simulink model "gm_Model"  (R2025a)
settings: Solver=FixedStepDiscrete  StartTime=0.0  StopTime=80000/fs_in  RelTol=1e-3
undefined symbols (not defined in the file or in its folder): a, b, b_fixp, beta_retanh, c, cos_omega, cos_omega_fixp, diag_count, exp_omega, exp_omega_fixp, fixp_chebacc_frac, fixp_chebacc_ws, fixp_dsp_ws, fixp_eig_frac, fixp_eig_ws, fs_in, group_size, hann_table_fixp, image_seed, image_seed_fixp, J_ROM, k, K_ROM, lap_diags, lap_main, lap_main_fi, lap_offsets, lap_offsets_fi, lap_rest, lap_rest_fi, laplacian_diags_main, laplacian_diags_offsets, laplacian_diags_rest, lut_norm_x, lut_norm_y, magnitude, n_ch, n_layer, n_px, n_px_fi, nf, norm_gain_floor, power_iters, power_norm_scaling_factor_fixp, tau, tau_fixp, theta, theta_fixp
libraries: simulink x59, hdlsllib x36, hdlstreaminglib x4, hdlmdlgenlib x1, matrix_library x1, dspvision x1
(part 3 of 8)

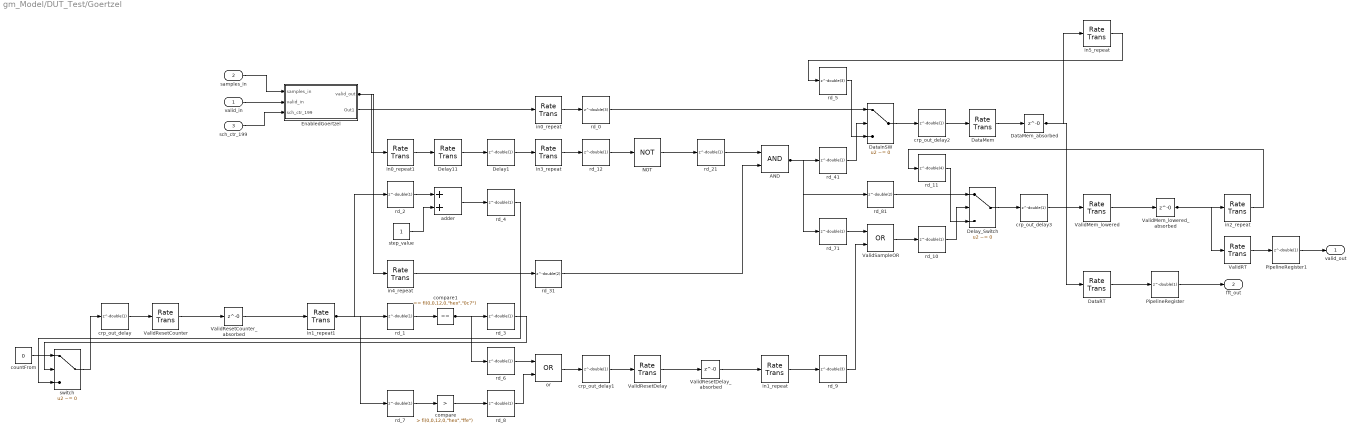
== system gm_Model/DUT_Test/Goertzel ==
  valid_in : Inport  OutDataTypeStr=boolean  PortDimensions=1  SampleTime=6.25e-05
  samples_in : Inport  Port=2  OutDataTypeStr=fixdt(1, 12, 11)  PortDimensions=[1 48]  SampleTime=6.25e-05
  sch_ctr_199 : Inport  Port=3  OutDataTypeStr=uint8  SampleTime=3.125e-07
  AND : Logic  AllPortsSameDT=off  OutDataTypeStr=boolean  SampleTime=3.125e-07
  DataInSW : Switch  Criteria=u2 ~= 0  Threshold="fi(0,0,1,0,\"hex\",\"0\")"  OutDataTypeStr=fixdt(1, 18, 13)  SampleTime=3.125e-07  SaturateOnIntegerOverflow=off  InputSameDT=off
  DataMem : RateTransition  InitialCondition=double(0)  OutPortSampleTimeOpt=Multiple of input port sample time  OutPortSampleTimeMultiple=200
  DataMem_absorbed : Delay  DelayLength=0
  DataRT : RateTransition  InitialCondition=double(0)  OutPortSampleTimeOpt=Multiple of input port sample time  OutPortSampleTimeMultiple=200
  Delay1 : Delay  DelayLength=double(1)  InitialCondition=0  SampleTime=6.25e-05
  Delay11 : RateTransition  InitialCondition=double(0)  OutPortSampleTimeOpt=Multiple of input port sample time  OutPortSampleTimeMultiple=200
  Delay_Switch : Switch  Criteria=u2 ~= 0  Threshold=double(0)  OutDataTypeStr=boolean  SampleTime=3.125e-07  SaturateOnIntegerOverflow=off  InputSameDT=off
  EnabledGoertzel : Subsystem
  NOT : Logic  Operator=NOT  Inputs=1  AllPortsSameDT=off  OutDataTypeStr=boolean  SampleTime=3.125e-07
  PipelineRegister : Delay  DelayLength=double(1)  InitialCondition=0  SampleTime=0.0125
  PipelineRegister1 : Delay  DelayLength=double(1)  InitialCondition=0  SampleTime=0.0125
  ValidMem_lowered : RateTransition  InitialCondition=double(0)  OutPortSampleTimeOpt=Multiple of input port sample time  OutPortSampleTimeMultiple=200
  ValidMem_lowered_absorbed : Delay  DelayLength=0
  ValidRT : RateTransition  InitialCondition=double(0)  OutPortSampleTimeOpt=Multiple of input port sample time  OutPortSampleTimeMultiple=200
  ValidResetCounter : RateTransition  InitialCondition=double(0)  OutPortSampleTimeOpt=Multiple of input port sample time  OutPortSampleTimeMultiple=200
  ValidResetCounter_absorbed : Delay  DelayLength=0
  ValidResetDelay : RateTransition  InitialCondition=double(0)  OutPortSampleTimeOpt=Multiple of input port sample time  OutPortSampleTimeMultiple=200
  ValidResetDelay_absorbed : Delay  DelayLength=0
  ValidSampleOR : Logic  Operator=OR  AllPortsSameDT=off  OutDataTypeStr=boolean  SampleTime=3.125e-07
  adder : Sum  OutDataTypeStr=fixdt(0, 12, 0)  AccumDataTypeStr=fixdt(0, 12, 0)  SampleTime=3.125e-07
  compare : simulink/Logic and Bit Operations/Compare To Constant  relop=>  const="fi(0,0,12,0,\"hex\",\"ffe\")"  OutDataTypeStr=boolean
  compare1 : simulink/Logic and Bit Operations/Compare To Constant  relop===  const="fi(0,0,12,0,\"hex\",\"0c7\")"  OutDataTypeStr=boolean
  countFrom : Constant  Value=0  VectorParams1D=off  OutDataTypeStr=fixdt(0, 12, 0)  SampleTime=3.125e-07
  crp_out_delay{,1..3} (4 alike) : Delay  DelayLength=double(1)  InitialCondition=0  SampleTime=3.125e-07
  in0_repeat : RateTransition  Integrity=off  Deterministic=off  OutPortSampleTimeOpt=Multiple of input port sample time  OutPortSampleTimeMultiple=1/200
  in0_repeat1 : RateTransition  Integrity=off  Deterministic=off  OutPortSampleTimeOpt=Multiple of input port sample time  OutPortSampleTimeMultiple=1/200
  in1_repeat : RateTransition  Integrity=off  Deterministic=off  OutPortSampleTimeOpt=Multiple of input port sample time  OutPortSampleTimeMultiple=1/200
  in1_repeat1 : RateTransition  Integrity=off  Deterministic=off  OutPortSampleTimeOpt=Multiple of input port sample time  OutPortSampleTimeMultiple=1/200
  in2_repeat : RateTransition  Integrity=off  Deterministic=off  OutPortSampleTimeOpt=Multiple of input port sample time  OutPortSampleTimeMultiple=1/200
  in3_repeat : RateTransition  Integrity=off  Deterministic=off  OutPortSampleTimeOpt=Multiple of input port sample time  OutPortSampleTimeMultiple=1/200
  in4_repeat : RateTransition  Integrity=off  Deterministic=off  OutPortSampleTimeOpt=Multiple of input port sample time  OutPortSampleTimeMultiple=1/200
  in5_repeat : RateTransition  Integrity=off  Deterministic=off  OutPortSampleTimeOpt=Multiple of input port sample time  OutPortSampleTimeMultiple=1/200
  or : Logic  Operator=OR  AllPortsSameDT=off  OutDataTypeStr=boolean  SampleTime=3.125e-07
  rd_0 : Delay  DelayLength=double(3)  InitialCondition=0  SampleTime=3.125e-07
  rd_{1..4,6..8,10,12,21,41,71} (12 alike) : Delay  DelayLength=double(1)  InitialCondition=0  SampleTime=3.125e-07
  rd_11 : Delay  DelayLength=double(4)  InitialCondition=0  SampleTime=3.125e-07
  rd_31 : Delay  DelayLength=double(2)  InitialCondition=0  SampleTime=3.125e-07
  rd_5 : Delay  DelayLength=double(3)  InitialCondition=0  SampleTime=3.125e-07
  rd_81 : Delay  DelayLength=double(2)  InitialCondition=0  SampleTime=3.125e-07
  rd_9 : Delay  DelayLength=double(3)  InitialCondition=0  SampleTime=3.125e-07
  step_value : Constant  VectorParams1D=off  OutDataTypeStr=fixdt(0, 12, 0)  SampleTime=3.125e-07
  switch : Switch  Criteria=u2 ~= 0  Threshold="fi(0,0,1,0,\"hex\",\"0\")"  OutDataTypeStr=fixdt(0, 12, 0)  SampleTime=3.125e-07  SaturateOnIntegerOverflow=off  InputSameDT=off
  valid_out : Outport  SampleTime=0.0125
  fft_out : Outport  Port=2  SampleTime=0.0125
  wires:
  valid_in/1 -> EnabledGoertzel/2(valid_in)
  countFrom/1 -> switch/1
  ValidResetDelay_absorbed/1 -> in1_repeat/1
  adder/1 -> rd_4/1
  switch/1 -> crp_out_delay/1
  in5_repeat/1 -> rd_5/1
  in1_repeat1/1 -> rd_2/1, rd_1/1, rd_7/1
  crp_out_delay/1 -> ValidResetCounter/1
  DataMem/1 -> DataMem_absorbed/1
  ValidResetCounter_absorbed/1 -> in1_repeat1/1
  DataMem_absorbed/1 -> DataRT/1, in5_repeat/1
  ValidResetCounter/1 -> ValidResetCounter_absorbed/1
  rd_0/1 -> DataInSW/1
  samples_in/1 -> EnabledGoertzel/1(samples_in)
  sch_ctr_199/1 -> EnabledGoertzel/3(sch_ctr_199)
  EnabledGoertzel/1(valid_out) -> in4_repeat/1, in0_repeat1/1
  DataInSW/1 -> crp_out_delay2/1
  EnabledGoertzel/2(Out1) -> in0_repeat/1
  in0_repeat1/1 -> Delay11/1
  rd_2/1 -> adder/1
  step_value/1 -> adder/2
  in4_repeat/1 -> rd_31/1
  ValidMem_lowered/1 -> ValidMem_lowered_absorbed/1
  rd_1/1 -> compare1/1
  PipelineRegister1/1 -> valid_out/1
  rd_7/1 -> compare/1
  Delay11/1 -> Delay1/1
  compare1/1 -> rd_6/1, rd_3/1
  compare/1 -> rd_8/1
  Delay1/1 -> in3_repeat/1
  or/1 -> crp_out_delay1/1
  rd_4/1 -> switch/3
  rd_3/1 -> switch/2
  rd_9/1 -> ValidSampleOR/2
  rd_8/1 -> or/2
  rd_6/1 -> or/1
  in3_repeat/1 -> rd_12/1
  in0_repeat/1 -> rd_0/1
  rd_31/1 -> AND/2
  rd_12/1 -> NOT/1
  crp_out_delay1/1 -> ValidResetDelay/1
  NOT/1 -> rd_21/1
  ValidResetDelay/1 -> ValidResetDelay_absorbed/1
  rd_81/1 -> Delay_Switch/1
  rd_21/1 -> AND/1
  AND/1 -> rd_71/1, rd_41/1, rd_81/1
  in1_repeat/1 -> rd_9/1
  rd_5/1 -> DataInSW/3
  ValidMem_lowered_absorbed/1 -> ValidRT/1, in2_repeat/1
  rd_41/1 -> DataInSW/2
  crp_out_delay2/1 -> DataMem/1
  rd_71/1 -> ValidSampleOR/1
  Delay_Switch/1 -> crp_out_delay3/1
  ValidSampleOR/1 -> rd_10/1
  rd_11/1 -> Delay_Switch/3
  rd_10/1 -> Delay_Switch/2
  DataRT/1 -> PipelineRegister/1
  crp_out_delay3/1 -> ValidMem_lowered/1
  ValidRT/1 -> PipelineRegister1/1
  PipelineRegister/1 -> fft_out/1
  in2_repeat/1 -> rd_11/1

== system gm_Model/DUT_ref/Backprojection ==
  valid_in : Inport
  In1 : Inport  Port=2
  For Each Subsystem : Subsystem  TreatAsAtomicUnit=on  mask{b=b, tau=tau}
  valid_out : Outport
  Out1 : Outport  Port=2
  wires:
  valid_in/1 -> valid_out/1
  For Each Subsystem/1(Out1) -> Out1/1
  In1/1 -> For Each Subsystem/1(In1)

== system gm_Model/DUT_ref/CrossCor ==
  valid_in : Inport
  data_in : Inport  Port=2
  Correlation : Subsystem
  Delay1 : Delay  DelayLength=1
  Grouping : Subsystem
  NormalizationEigen : Subsystem  Commented=on
  NormalizationPower : Subsystem
  valid_out : Outport
  data_out : Outport  Port=2
  wires:
  NormalizationPower/1(data_out) -> data_out/1
  Delay1/1 -> valid_out/1
  Grouping/1(valid) -> Delay1/1
  Grouping/2(out) -> NormalizationEigen/1(In1), NormalizationPower/1(out)
  valid_in/1 -> Grouping/1(en)
  Correlation/1(in) -> Grouping/2(in)
  data_in/1 -> Correlation/1(In1)

== system gm_Model/DUT_ref/Deblurring ==
  note: Chebyshev also verified to work correctly!
      | Very slight difference (<0.0003), possibly due to FP rounding errors?
      | (Different way of calculating compared to Python)
  valid_in : Inport
  Image_in : Inport  Port=2
  Cheb_out : Selector  Commented=on  InputPortWidth=n_px  IndexOptions=Index vector (dialog)  Indices=1  OutputSizes=1
  Chebyshev : Subsystem
  Chev_in : Selector  Commented=on  InputPortWidth=n_px  IndexOptions=Index vector (dialog)  Indices=1  OutputSizes=1
  Delay : Delay  DelayLength=1
  Delay2 : Delay  DelayLength=1
  Gain : Gain  Gain=beta_retanh
  ImageInFast : Selector  Commented=on  InputPortWidth=n_px  IndexOptions=Index vector (dialog)  Indices=1  OutputSizes=1
  ImageInSlow : Selector  Commented=on  InputPortWidth=n_px  IndexOptions=Index vector (dialog)  Indices=1  OutputSizes=1
  ImageSeed : Constant  Value=image_seed  SampleTime=-1
  LayerCounter : hdlsllib/Sources/HDL Counter  CountType=Count limited  CountInit=0  CountStep=1  CountMax=n_layer-1  CountFromType=Initial value  CountFrom=0  CountResetPort=off  CountLoadPort=off  CountEnbPort=off  CountDirPort=off  CountHitOutputPort=on  CountDataType=Unsigned  CountWordLen=6  CountFracLen=0  CountSampTime=-1
  Max : MinMax  Function=max  Inputs=2
  Rate Transition : RateTransition  Integrity=off  Deterministic=off  OutPortSampleTimeOpt=Multiple of input port sample time  OutPortSampleTimeMultiple=1/n_layer  OutPortSampleTime=n_layer
  Rate Transition1 : RateTransition  Integrity=off  Deterministic=off  OutPortSampleTimeOpt=Multiple of input port sample time  OutPortSampleTimeMultiple=1/n_layer  OutPortSampleTime=n_layer
  Rate Transition2 : RateTransition  OutPortSampleTimeOpt=Multiple of input port sample time  OutPortSampleTimeMultiple=n_layer  OutPortSampleTime=n_layer
  Rate Transition3 : RateTransition  OutPortSampleTimeOpt=Multiple of input port sample time  OutPortSampleTimeMultiple=n_layer  OutPortSampleTime=n_layer
  Sum : Sum  Inputs=++|
  Switch : Switch  Criteria=u2 > Threshold  SaturateOnIntegerOverflow=off  InputSameDT=off
  Tanh : Trigonometry  Operator=tanh
  To Workspace : ToWorkspace  Commented=on  VariableName=image_in  SaveFormat=Timeseries  SampleTime=-1
  To Workspace1 : ToWorkspace  Commented=on  VariableName=image_out  SaveFormat=Timeseries  SampleTime=-1
  Zero : Constant  Value=0  OutDataTypeStr=Inherit: Inherit via back propagation  SampleTime=-1
  valid_out : Outport
  Out1 : Outport  Port=2
  wires:
  Max/1 -> Switch/1, Rate Transition3/1
  Zero/1 -> Max/2
  Gain/1 -> Max/1
  Delay/1 -> Rate Transition2/1
  Switch/1 -> To Workspace/1, Chebyshev/1(Image_in), Chev_in/1
  Chebyshev/1(Out1) -> Sum/2, To Workspace1/1, Cheb_out/1
  ImageSeed/1 -> Switch/3
  Delay2/1 -> Sum/1
  Rate Transition3/1 -> Out1/1
  Rate Transition2/1 -> valid_out/1  "ValidOutSlow"
  Rate Transition1/1 -> Delay/1  "ValidInFast"
  valid_in/1 -> Rate Transition1/1  "ValidInSlow"
  Rate Transition/1 -> Delay2/1, ImageInFast/1
  Sum/1 -> Tanh/1
  Image_in/1 -> ImageInSlow/1, Rate Transition/1
  Tanh/1 -> Gain/1
  LayerCounter/1 -> Switch/2

== system gm_Model/DUT_ref/Goertzel ==
  valid_in : Inport
  In1 : Inport  Port=2
  DataValidDownsampler : Subsystem
  EnabledGoertzel : Subsystem
  GoertzelOutInt : Selector  Commented=on  InputPortWidth=48  IndexOptions=Index vector (dialog)  Indices=1  OutputSizes=1
  GoertzelOutSlow : Selector  Commented=on  InputPortWidth=48  IndexOptions=Index vector (dialog)  Indices=1  OutputSizes=1
  State Control : StateControl  StateControl=Synchronous
  valid_out : Outport
  DataSlow : Outport  Port=2
  wires:
  DataValidDownsampler/2(DataSlow) -> GoertzelOutSlow/1, DataSlow/1
  DataValidDownsampler/1(ValidSlow) -> valid_out/1
  EnabledGoertzel/1(valid_out) -> DataValidDownsampler/1(ValidFast)
  EnabledGoertzel/2(Out1) -> GoertzelOutInt/1, DataValidDownsampler/2(DataFast)
  valid_in/1 -> EnabledGoertzel/Enable
  In1/1 -> EnabledGoertzel/1(In2)

== system gm_Model/Unused blocks/BackprojOpt ==
  In1 : Inport
  Constant : Constant  Value=b  SampleTime=-1
  Constant1 : Constant  Value=tau
  Dot Product : DotProduct  OutDataTypeStr=Inherit: Inherit via internal rule
  For Each : ForEach  DisableCoverage=on  IterateSubsysMaskParameter=on,on  SubsysMaskParameterIterationDimension=2,2
  For Each Subsystem : Subsystem  Commented=on  TreatAsAtomicUnit=on  mask{K=K_ROM, J=J_ROM}
  MATLAB Function : MATLAB Function  TreatAsAtomicUnit=on
  Magnitude Squared : Math  Operator=magnitude^2
  ShiftBy2 : Gain  Gain=2
  Sum : Sum  Inputs=-++
  Sum of Elements : Sum  Inputs=+
  Out1 : Outport  ConcatenationDimension=1
  wires:
  ShiftBy2/1 -> Sum/3
  Sum of Elements/1 -> ShiftBy2/1
  For Each Subsystem/1(Out1) -> Sum of Elements/1
  MATLAB Function/1(y) -> Dot Product/2
  In1/1 -> MATLAB Function/1(A), For Each Subsystem/1(cc)
  Magnitude Squared/1 -> Dot Product/1
  Constant/1 -> Magnitude Squared/1, For Each Subsystem/2(b)
  Sum/1 -> Out1/1
  Dot Product/1 -> Sum/2
  Constant1/1 -> Sum/1

== system gm_Model/Unused blocks/For Each Subsystem ==
  note: Main Diagonal
  ToIterate : Inport  Partition=on  PartitionDimension=1  PartitionWidth=1  PartitionOffset=0
  Image : Inport  Port=2
  Cast : DataTypeConversion  OutDataTypeStr=fixdt(0,ceil(log2(n_px)),0)  SaturateOnIntegerOverflow=off  RndMeth=Floor
  For Each : ForEach  DisableCoverage=on  ShowIterationIndex=on
  MainDiagonal : MATLAB Function  TreatAsAtomicUnit=on
  Terminator : Terminator
  Image_out : Outport  ConcatenationDimension=1
  wires:
  MainDiagonal/1(out) -> Image_out/1
  Cast/1 -> MainDiagonal/2(index)
  For Each/1 -> Cast/1
  ToIterate/1 -> Terminator/1
  Image/1 -> MainDiagonal/1(image_in)

== system gm_Model/DUT_FixP/Backprojection/BackprojNaive ==
  In1 : Inport
  Complex to Real-Imag : ComplexToRealImag  Output=Real
  Constant : Constant  Value=b  SampleTime=-1
  Constant1 : Constant  Value=tau  SampleTime=-1
  Delay : Delay  DelayLength=1
  Delay1 : Delay  DelayLength=1
  Delay2 : Delay  DelayLength=1
  For Each : ForEach  DisableCoverage=on  IterateSubsysMaskParameter=on,on  SubsysMaskParameterIterationDimension=2,2
  Hermitian : Math  Operator=hermitian
  Matrix Multiply : Product  Multiplication=Matrix(*)  OutDataTypeStr=fixdt(1,fixp_bpp_ws,fixp_bpp_frac)
  Matrix Multiply1 : Product  Multiplication=Matrix(*)  OutDataTypeStr=fixdt(1,fixp_dbl_ws,fixp_dbl_frac)
  Sum : Sum  Inputs=|+-  OutDataTypeStr=Inherit: Same as accumulator
  Out1 : Outport  ConcatenationDimension=1
  wires:
  Delay2/1 -> Out1/1
  Delay1/1 -> Matrix Multiply1/2
  Delay/1 -> Matrix Multiply1/1
  Sum/1 -> Delay2/1
  Constant/1 -> Delay1/1, Hermitian/1
  Constant1/1 -> Sum/2
  Complex to Real-Imag/1 -> Sum/1
  In1/1 -> Matrix Multiply/2
  Matrix Multiply1/1 -> Complex to Real-Imag/1
  Matrix Multiply/1 -> Delay/1
  Hermitian/1 -> Matrix Multiply/1

== system gm_Model/DUT_FixP/CrossCor/Correlation ==
  In1 : Inport
  Delay : Delay  DelayLength=1
  Math Function1 : Math  Operator=hermitian
  MatrixMultiply : Product  Multiplication=Matrix(*)  OutDataTypeStr=Inherit: Same as first input
  in : Outport
  wires:
  Delay/1 -> in/1
  In1/1 -> Math Function1/1, MatrixMultiply/2
  Math Function1/1 -> MatrixMultiply/1
  MatrixMultiply/1 -> Delay/1

== system gm_Model/DUT_FixP/CrossCor/Grouping ==
  note: Sum 9 frames and reduce data rate
  valid_in : Inport
  in : Inport  Port=2
  Add : Sum  OutDataTypeStr=Inherit: Same as accumulator  AccumDataTypeStr=fixdt(1,fixp_input_ws+fixp_goertzel_int_bits+2,fixp_input_ws+2-1)
  DataValidDownsampler : Subsystem  mask{rate_factor=group_size}
  Delay : Delay  DelayLength=1
  Delay1 : Delay  DelayLength=1
  HDL Counter : hdlsllib/Sources/HDL Counter  CountType=Count limited  CountInit=0  CountStep=1  CountMax=group_size-1  CountFromType=Initial value  CountFrom=0  CountResetPort=off  CountLoadPort=off  CountEnbPort=on  CountDirPort=off  CountHitOutputPort=on  CountDataType=Unsigned  CountWordLen=ceil(log2(group_size))  CountFracLen=0  CountSampTime=-1
  Real-Imag to Complex : RealImagToComplex
  Real-Imag to Complex1 : RealImagToComplex
  Switch : Switch  Criteria=u2 ~= 0  SaturateOnIntegerOverflow=off  InputSameDT=off
  Switch1 : Switch  Criteria=u2 ~= 0  SaturateOnIntegerOverflow=off  InputSameDT=off
  Terminator : Terminator
  Zero : Constant  Value=0  OutDataTypeStr=Inherit: Inherit via back propagation  SampleTime=-1
  Zero1 : Constant  Value=0  OutDataTypeStr=Inherit: Inherit via back propagation  SampleTime=-1
  valid : Outport
  out : Outport  Port=2
  wires:
  DataValidDownsampler/1(ValidSlow) -> valid/1
  DataValidDownsampler/2(DataSlow) -> out/1
  HDL Counter/1 -> Terminator/1
  Real-Imag to Complex1/1 -> Switch1/3
  Zero1/1 -> Real-Imag to Complex1/1, Real-Imag to Complex1/2
  in/1 -> Switch1/1
  Switch1/1 -> Add/1
  valid_in/1 -> HDL Counter/1, Switch1/2
  Real-Imag to Complex/1 -> Switch/1
  Switch/1 -> Add/2
  Delay/1 -> DataValidDownsampler/2(DataFast), Switch/3
  Add/1 -> Delay/1
  Delay1/1 -> Switch/2, DataValidDownsampler/1(ValidFast)
  Zero/1 -> Real-Imag to Complex/1, Real-Imag to Complex/2
  HDL Counter/2 -> Delay1/1

== system gm_Model/DUT_FixP/CrossCor/NormalizationEig ==
  valid_in : Inport
  out : Inport  Port=2
      settings: SignalType=complex
  Constant : Constant  Value=1+2^-fixp_eig_frac  OutDataTypeStr=Inherit: Inherit via back propagation  SampleTime=-1
  Delay : Delay  DelayLength=1
  Delay1 : Delay
  Delay2 : Delay  DelayLength=1
  Delay3 : Delay  DelayLength=1
  EigReciprocalLUT : Lookup_n-D  Commented=on  NumberOfTableDimensions=1  LookupTableObject=FSds  BreakpointsForDimension1=lut_norm_x  BreakpointsForDimension1FirstPoint=10  BreakpointsForDimension2FirstPoint=10  BreakpointsForDimension1Spacing=12  BreakpointsForDimension2Spacing=12  BreakpointsForDimension1DataTypeStr=Inherit: Inherit from 'Breakpoint data'  Table=lut_norm_y  TableDataTypeStr=Inherit: Inherit from 'Table data'  ExtrapMethod=Clip  DiagnosticForOutOfRangeInput=Error  RemoveProtectionInput=on  UseLastTableValue=on  OutDataTypeStr=Inherit: Inherit from 'Table data'  RndMeth=Simplest
  Max : MinMax  Function=max  Inputs=2
  PowerIteration : Subsystem
  Product : Product  OutDataTypeStr=Inherit: Same as first input
  Reciprocal : Product  Inputs=/  OutDataTypeStr=fixdt(0,24,23)
  valid_out : Outport
  data_out : Outport  Port=2
  Eig_value : Outport  Port=3
  wires:
  Reciprocal/1 -> Product/2
  Max/1 -> Reciprocal/1, EigReciprocalLUT/1
  Delay3/1 -> Eig_value/1
  Delay2/1 -> data_out/1
  Delay/1 -> valid_out/1
  valid_in/1 -> Delay1/1
  Delay1/1 -> Delay/1
  out/1 -> PowerIteration/1(MatIn)
  PowerIteration/2(MaxEigenvalue) -> Delay3/1, Max/1
  Constant/1 -> Max/2
  PowerIteration/1(MatOut) -> Product/1
  Product/1 -> Delay2/1

== system gm_Model/DUT_FixP/CrossCor/NormalizationPower ==
  valid_in : Inport
  out : Inport  Port=2
      settings: SignalType=complex
  Complex to Real-Imag : ComplexToRealImag  Output=Real
  Constant : Constant  Value=1+2^-fixp_eig_frac  OutDataTypeStr=Inherit: Inherit via back propagation  SampleTime=-1
  Delay : Delay  DelayLength=1
  Delay1 : Delay  DelayLength=1
  Delay2 : Delay  DelayLength=1
  Diag : MATLAB Function  TreatAsAtomicUnit=on
  Gain : Gain  Gain=power_norm_scaling_factor_fixp  ParamDataTypeStr=Inherit: Inherit from 'Gain'  OutDataTypeStr=Inherit: Same as input
  Max1 : MinMax  Function=max  Inputs=2
  Product : Product  OutDataTypeStr=Inherit: Same as first input
  Reciprocal : Product  Inputs=/  OutDataTypeStr=fixdt(0,24,23)  SaturateOnIntegerOverflow=on
  Sum of Elements : Sum  Inputs=+
  valid_out : Outport
  data_out : Outport  Port=2
  norm_out : Outport  Port=3
  wires:
  Max1/1 -> Reciprocal/1
  Constant/1 -> Max1/2
  Gain/1 -> Max1/1, Delay1/1
  Delay1/1 -> norm_out/1
  Complex to Real-Imag/1 -> Sum of Elements/1
  Diag/1(y) -> Complex to Real-Imag/1
  Reciprocal/1 -> Product/2
  Sum of Elements/1 -> Gain/1
  Delay2/1 -> data_out/1
  Delay/1 -> valid_out/1
  valid_in/1 -> Delay/1
  out/1 -> Product/1, Diag/1(u)
  Product/1 -> Delay2/1

== system gm_Model/DUT_FixP/Deblurring/Chebyshev ==
  note: In to output delay (in slow IO speed): 1
  Image_in : Inport
  AccumulatorCounter : Subsystem
  Constant1 : Constant  Value=theta_fixp  SampleTime=-1
  Delay2 : Delay
  Gain1 : Gain  Gain=2  OutDataTypeStr=Inherit: Same as input
  Index Vector : MultiPortSwitch  DataPortOrder=Zero-based contiguous  DiagnosticForDefault=None  zeroidx=on  SaturateOnIntegerOverflow=off  InputSameDT=off
  LaplacianMultiply : Subsystem
  MakeSigned : DataTypeConversion  OutDataTypeStr=fixdt(1,fixp_lapmult_ws,fixp_lapmult_frac)  SaturateOnIntegerOverflow=off  RndMeth=Floor
  Rate Transition : RateTransition  Integrity=off  OutPortSampleTimeOpt=Multiple of input port sample time  OutPortSampleTimeMultiple=1/(k+1)
  Rate Transition2 : RateTransition  OutPortSampleTimeOpt=Multiple of input port sample time  OutPortSampleTimeMultiple=k+1
  Selector1 : Selector  IndexMode=Zero-based  InputPortWidth=k+1  IndexOptions=Index vector (port)  Indices=[1 3]  OutputSizes=1
  Sum1 : Sum  Inputs=|+-  OutDataTypeStr=Inherit: Same as accumulator
  Out1 : Outport
  wires:
  MakeSigned/1 -> Index Vector/2
  Rate Transition/1 -> MakeSigned/1
  LaplacianMultiply/1(Image_out) -> Index Vector/3, Gain1/1
  [cheb_iter] -> Selector1/2
  AccumulatorCounter/1(counter) -> [cheb_iter]
  Constant1/1 -> Selector1/1
  Rate Transition2/1 -> Out1/1
  AccumulatorCounter/2(accum) -> Rate Transition2/1
  Selector1/1 -> AccumulatorCounter/1(a)
  [cheb_iter] -> Index Vector/1
  Image_in/1 -> Rate Transition/1
  Index Vector/1 -> AccumulatorCounter/2(b), Delay2/1, LaplacianMultiply/1(Image_in)  "z_k"
  Sum1/1 -> Index Vector/4
  Delay2/1 -> Sum1/2  "z_k-2"
  Gain1/1 -> Sum1/1

== system gm_Model/DUT_FixP/Goertzel/DataValidDownsampler ==
  ValidFast : Inport
  DataFast : Inport  Port=2
  DataInSW : Switch  Criteria=u2 ~= 0  SaturateOnIntegerOverflow=off  InputSameDT=off
  DataMem : Delay  DelayLength=1
  DataRT : RateTransition  OutPortSampleTimeOpt=Multiple of input port sample time  OutPortSampleTimeMultiple=nf
  RisingEdgeDetector : Subsystem
  Terminator : Terminator
  ValidMem : Delay  DelayLength=1  ShowEnablePort=on
      settings: InputPortMap=u0,e6
  ValidRT : RateTransition  OutPortSampleTimeOpt=Multiple of input port sample time  OutPortSampleTimeMultiple=nf
  ValidResetCounter : hdlsllib/Sources/HDL Counter  CountType=Count limited  CountInit=0  CountStep=1  CountMax=nf-1  CountFromType=Initial value  CountFrom=0  CountResetPort=off  CountLoadPort=off  CountEnbPort=off  CountDirPort=off  CountHitOutputPort=on  CountDataType=Unsigned  CountWordLen=12  CountFracLen=0  CountSampTime=-1
  ValidResetDelay : Delay  DelayLength=1
  ValidSampleOR : Logic  Operator=OR  IconShape=distinctive  AllPortsSameDT=off  OutDataTypeStr=boolean
  ValidSlow : Outport
  DataSlow : Outport  Port=2
  wires:
  ValidResetCounter/1 -> Terminator/1
  DataFast/1 -> DataInSW/1
  DataRT/1 -> DataSlow/1
  ValidRT/1 -> ValidSlow/1
  ValidMem/1 -> ValidRT/1
  ValidResetDelay/1 -> ValidSampleOR/2
  ValidResetCounter/2 -> ValidResetDelay/1
  ValidFast/1 -> RisingEdgeDetector/1(In1)
  RisingEdgeDetector/1(Out1) -> ValidMem/1, ValidSampleOR/1, DataInSW/2
  DataInSW/1 -> DataMem/1
  DataMem/1 -> DataInSW/3, DataRT/1
  ValidSampleOR/1 -> ValidMem/2

== system gm_Model/DUT_FixP/Goertzel/EnabledGoertzel ==
  samples_in : Inport
  valid_in : EnablePort
  Delay : Delay
  Delay{1..4} (4 alike) : Delay  DelayLength=1
  Goertzel filter : Subsystem  TreatAsAtomicUnit=on
      settings: PortSchema="{\"entries\":[{\"content\":{\"sides\":[{\"content\":{\"connectorIds\":[\"In1\"]},\"type\":\"ConnectorPlacement.EquallySpacedRectSide\",\"uuid\":\"8ecbe949-c7a4-4917-b668-844d41a795fc\"},{\"content\":{\"connectorIds\":[\"Out1\"],\"side\":\"RIGHT\"},\"type\":\"ConnectorPlacement.EquallySpacedRectSide\",\"uuid\":\"beb6ac4b-4365-4b4a-bc98-03b942c90e20\"},{\"content\":{\"connectorIds\":[\"In2\"],\"side\":\"TOP\"},\"type\":\"ConnectorPlacement.EquallySpacedRectSide\",\"uuid\":\"0b5f67b8-767c-4b8f-bb43-2f6787e0e6b5\"}]},\"type\":\"ConnectorPlacement.EquallySpacedConnector\",\"uuid\":\"125f6c5b-451b-4cfb-80b8-61098e2de1e6\"}],\"packageUris\":[\"http://schema.mathworks.com/mf0/Connector/R2020b\"],\"version\":\"1.0\"}"
  HDL Counter : hdlsllib/Sources/HDL Counter  CountType=Count limited  CountInit=0  CountStep=1  CountMax=nf-1  CountFromType=Initial value  CountFrom=0  CountResetPort=off  CountLoadPort=off  CountEnbPort=off  CountDirPort=off  CountHitOutputPort=on  CountDataType=Unsigned  CountWordLen=8  CountFracLen=0  CountSampTime=1/fs_in
  Product : Product  OutDataTypeStr=fixdt(1,fixp_input_ws+2,fixp_input_ws+1)
  Symmetric Hann : Subsystem
  valid_out : Outport
  Out1 : Outport  Port=2
  wires:
  Delay4/1 -> valid_out/1
  Delay3/1 -> Out1/1
  Delay2/1 -> Symmetric Hann/1(u)
  Delay1/1 -> Product/2
  Delay/1 -> Goertzel filter/2(Reset), Delay4/1
  Goertzel filter/1(Out1) -> Delay3/1
  samples_in/1 -> Delay1/1
  Symmetric Hann/1(Out1) -> Product/1
  Product/1 -> Goertzel filter/1(u)
  HDL Counter/1 -> Delay2/1
  HDL Counter/2 -> Delay/1

== system gm_Model/DUT_Test/CrossCor/Reciprocal ==
  In1 : Inport
  Reciprocal : Product  Inputs=/  OutDataTypeStr=fixdt(0,24,23)  SaturateOnIntegerOverflow=on
  Reciprocal_pd1 : Delay  DelayLength=42
  Out1 : Outport
  wires:
  In1/1 -> Reciprocal/1
  Reciprocal/1 -> Reciprocal_pd1/1
  Reciprocal_pd1/1 -> Out1/1

== system gm_Model/DUT_Test/CrossCor/streaming_partition_streamed ==
  in0 : Inport  OutDataTypeStr=fixdt(0, 24, 23)  SampleTime=3.125e-07
  in1 : Inport  Port=2  OutDataTypeStr=fixdt(1, 18, 13)  PortDimensions=[2304 1]  SampleTime=3.125e-07
      settings: SignalType=complex
  enb_counter : Inport  Port=3  OutDataTypeStr=fixdt(0, 19, 0)  SampleTime=3.125e-07
  HwModeRegister{,1..3} (4 alike) : Delay  DelayLength=double(1)  InitialCondition=0  SampleTime=3.125e-07
  PipelineRegister : Delay  DelayLength=double(1)  InitialCondition=0  SampleTime=3.125e-07
  PipelineRegister1 : Delay  DelayLength=double(1)  InitialCondition=0  SampleTime=3.125e-07
  Product : Product  Inputs=**  OutDataTypeStr=fixdt(1, 18, 13)  SampleTime=3.125e-07
  Product1 : Product  Inputs=**  OutDataTypeStr=fixdt(1, 18, 13)  SampleTime=3.125e-07
  Product_C2ReIm : ComplexToRealImag  SampleTime=3.125e-07
  Product_ReIm2Complex : RealImagToComplex  SampleTime=3.125e-07
  Serializer_Subnetwork : Subsystem
  c3_Product_out1_bypass : Subsystem
  counter : Subsystem
  enb_counter_eq_49 : simulink/Logic and Bit Operations/Compare To Constant  relop===  const=double(49)  OutDataTypeStr=boolean
  enb_counter_ge_2 : simulink/Logic and Bit Operations/Compare To Constant  relop=>=  const=double(2)  OutDataTypeStr=boolean
  enb_counter_ge_2_and_enb_counter_le_48 : Logic  AllPortsSameDT=off  OutDataTypeStr=boolean  SampleTime=3.125e-07
  enb_counter_le_47 : simulink/Logic and Bit Operations/Compare To Constant  relop=<=  const=double(47)  OutDataTypeStr=boolean
  enb_counter_le_48 : simulink/Logic and Bit Operations/Compare To Constant  relop=<=  const=double(48)  OutDataTypeStr=boolean
  rd_{0..6} (7 alike) : Delay  DelayLength=double(1)  InitialCondition=0  SampleTime=3.125e-07
  rd_7 : Delay  DelayLength=double(2)  InitialCondition=0  SampleTime=3.125e-07
  t : Mux  Inputs=2
  tappedDelay : Subsystem
  out0 : Outport  OutDataTypeStr=fixdt(1, 18, 13)  PortDimensions=[2304 1]  SampleTime=3.125e-07
      settings: SignalType=complex
  wires:
  rd_0/1 -> counter/Enable
  enb_counter/1 -> enb_counter_le_48/1, enb_counter_eq_49/1, enb_counter_ge_2/1, enb_counter_le_47/1
  rd_4/1 -> enb_counter_ge_2_and_enb_counter_le_48/2
  enb_counter_le_48/1 -> rd_4/1
  rd_5/1 -> t/1
  tappedDelay/1(out0) -> rd_5/1
  enb_counter_ge_2/1 -> rd_3/1
  rd_3/1 -> enb_counter_ge_2_and_enb_counter_le_48/1
  enb_counter_le_47/1 -> rd_0/1
  PipelineRegister/1 -> Product_ReIm2Complex/2
  enb_counter_ge_2_and_enb_counter_le_48/1 -> tappedDelay/Enable
  in1/1 -> Serializer_Subnetwork/1(in0)
  counter/1(out0) -> Serializer_Subnetwork/2(in1)
  rd_7/1 -> c3_Product_out1_bypass/2(in1)
  Serializer_Subnetwork/1(out0) -> Product_C2ReIm/1
  in0/1 -> rd_1/1, rd_2/1
  enb_counter_eq_49/1 -> rd_7/1
  Product_C2ReIm/1 -> HwModeRegister2/1
  Product_C2ReIm/2 -> HwModeRegister/1
  rd_1/1 -> HwModeRegister3/1
  rd_2/1 -> HwModeRegister1/1
  HwModeRegister2/1 -> Product1/1
  HwModeRegister3/1 -> Product1/2
  Product1/1 -> PipelineRegister1/1
  HwModeRegister/1 -> Product/1
  HwModeRegister1/1 -> Product/2
  Product/1 -> PipelineRegister/1
  PipelineRegister1/1 -> Product_ReIm2Complex/1
  Product_ReIm2Complex/1 -> rd_6/1, tappedDelay/1(in0)
  rd_6/1 -> c3_Product_out1_bypass/1(in0)
  c3_Product_out1_bypass/1(out0) -> t/2
  t/1 -> out0/1

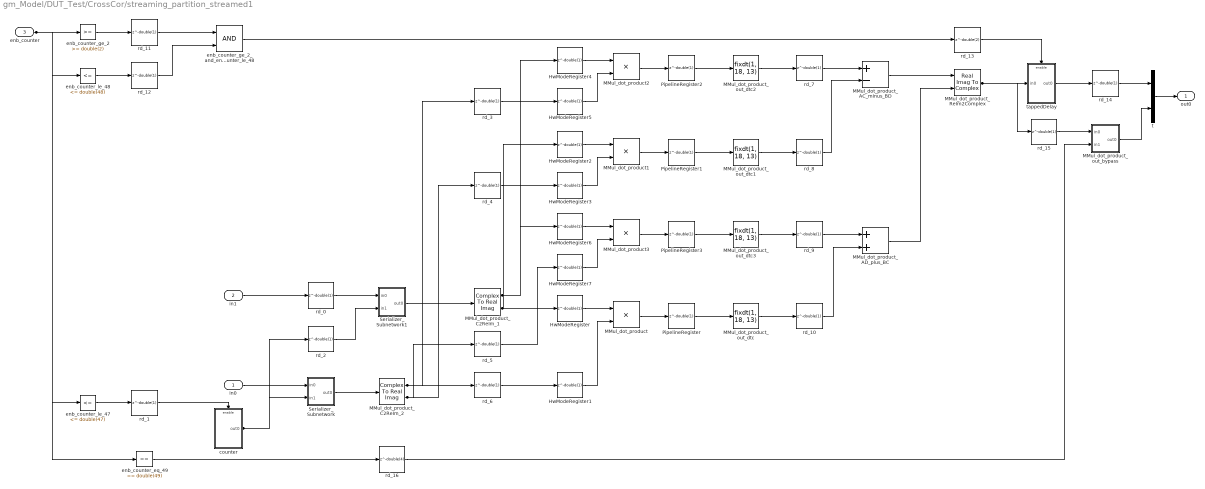
== system gm_Model/DUT_Test/CrossCor/streaming_partition_streamed1 ==
  in0 : Inport  OutDataTypeStr=fixdt(1, 18, 13)  PortDimensions=[2304 1]  SampleTime=3.125e-07
      settings: SignalType=complex
  in1 : Inport  Port=2  OutDataTypeStr=fixdt(1, 18, 13)  PortDimensions=[2304 1]  SampleTime=3.125e-07
      settings: SignalType=complex
  enb_counter : Inport  Port=3  OutDataTypeStr=uint16  SampleTime=3.125e-07
  HwModeRegister{,1..7} (8 alike) : Delay  DelayLength=double(1)  InitialCondition=0  SampleTime=3.125e-07
  MMul_dot_product{,1..3} (4 alike) : Product  Inputs=**  OutDataTypeStr=fixdt(1, 36, 26)  SampleTime=3.125e-07
  MMul_dot_product_AC_minus_BD : Sum  Inputs=+-  OutDataTypeStr=fixdt(1, 18, 13)  SampleTime=3.125e-07
  MMul_dot_product_AD_plus_BC : Sum  OutDataTypeStr=fixdt(1, 18, 13)  SampleTime=3.125e-07
  MMul_dot_product_C2ReIm_1 : ComplexToRealImag  SampleTime=3.125e-07
  MMul_dot_product_C2ReIm_2 : ComplexToRealImag  SampleTime=3.125e-07
  MMul_dot_product_ReIm2Complex : RealImagToComplex  SampleTime=3.125e-07
  MMul_dot_product_out_bypass : Subsystem
  MMul_dot_product_out_dtc{,1..3} (4 alike) : DataTypeConversion  OutDataTypeStr=fixdt(1, 18, 13)  SampleTime=3.125e-07  SaturateOnIntegerOverflow=off  RndMeth=Floor
  PipelineRegister{,1..3} (4 alike) : Delay  DelayLength=double(1)  InitialCondition=0  SampleTime=3.125e-07
  Serializer_Subnetwork : Subsystem
  Serializer_Subnetwork1 : Subsystem
  counter : Subsystem
  enb_counter_eq_49 : simulink/Logic and Bit Operations/Compare To Constant  relop===  const=double(49)  OutDataTypeStr=boolean
  enb_counter_ge_2 : simulink/Logic and Bit Operations/Compare To Constant  relop=>=  const=double(2)  OutDataTypeStr=boolean
  enb_counter_ge_2_and_enb_counter_le_48 : Logic  AllPortsSameDT=off  OutDataTypeStr=boolean  SampleTime=3.125e-07
  enb_counter_le_47 : simulink/Logic and Bit Operations/Compare To Constant  relop=<=  const=double(47)  OutDataTypeStr=boolean
  enb_counter_le_48 : simulink/Logic and Bit Operations/Compare To Constant  relop=<=  const=double(48)  OutDataTypeStr=boolean
  rd_{0..12,14..15} (15 alike) : Delay  DelayLength=double(1)  InitialCondition=0  SampleTime=3.125e-07
  rd_13 : Delay  DelayLength=double(2)  InitialCondition=0  SampleTime=3.125e-07
  rd_16 : Delay  DelayLength=double(4)  InitialCondition=0  SampleTime=3.125e-07
  t : Mux  Inputs=2
  tappedDelay : Subsystem
  out0 : Outport  OutDataTypeStr=fixdt(1, 18, 13)  PortDimensions=[2304 1]  SampleTime=3.125e-07
      settings: SignalType=complex
  wires:
  enb_counter/1 -> enb_counter_eq_49/1, enb_counter_le_48/1, enb_counter_ge_2/1, enb_counter_le_47/1
  MMul_dot_product/1 -> PipelineRegister/1
  enb_counter_ge_2/1 -> rd_11/1
  counter/1(out0) -> rd_2/1, Serializer_Subnetwork/2(in1)
  rd_11/1 -> enb_counter_ge_2_and_enb_counter_le_48/1
  enb_counter_le_48/1 -> rd_12/1
  enb_counter_eq_49/1 -> rd_16/1
  MMul_dot_product_out_dtc2/1 -> rd_7/1
  enb_counter_le_47/1 -> rd_1/1
  rd_12/1 -> enb_counter_ge_2_and_enb_counter_le_48/2
  rd_16/1 -> MMul_dot_product_out_bypass/2(in1)
  Serializer_Subnetwork1/1(out0) -> MMul_dot_product_C2ReIm_1/1
  rd_1/1 -> counter/Enable
  enb_counter_ge_2_and_enb_counter_le_48/1 -> rd_13/1
  rd_8/1 -> MMul_dot_product_AC_minus_BD/2
  rd_2/1 -> Serializer_Subnetwork1/2(in1)
  in1/1 -> rd_0/1
  in0/1 -> Serializer_Subnetwork/1(in0)
  rd_10/1 -> MMul_dot_product_AD_plus_BC/2
  rd_0/1 -> Serializer_Subnetwork1/1(in0)
  MMul_dot_product_out_dtc3/1 -> rd_9/1
  HwModeRegister5/1 -> MMul_dot_product2/2
  HwModeRegister4/1 -> MMul_dot_product2/1
  Serializer_Subnetwork/1(out0) -> MMul_dot_product_C2ReIm_2/1
  MMul_dot_product_C2ReIm_2/2 -> rd_4/1, rd_5/1
  MMul_dot_product_C2ReIm_2/1 -> rd_3/1, rd_6/1
  rd_5/1 -> HwModeRegister7/1
  rd_3/1 -> HwModeRegister5/1
  rd_4/1 -> HwModeRegister3/1
  MMul_dot_product3/1 -> PipelineRegister3/1
  MMul_dot_product_C2ReIm_1/1 -> HwModeRegister4/1, HwModeRegister6/1
  HwModeRegister6/1 -> MMul_dot_product3/1
  MMul_dot_product_C2ReIm_1/2 -> HwModeRegister/1, HwModeRegister2/1
  MMul_dot_product_out_dtc/1 -> rd_10/1
  rd_6/1 -> HwModeRegister1/1
  PipelineRegister1/1 -> MMul_dot_product_out_dtc1/1
  HwModeRegister2/1 -> MMul_dot_product1/1
  MMul_dot_product_ReIm2Complex/1 -> rd_15/1, tappedDelay/1(in0)
  HwModeRegister3/1 -> MMul_dot_product1/2
  HwModeRegister7/1 -> MMul_dot_product3/2
  MMul_dot_product_AC_minus_BD/1 -> MMul_dot_product_ReIm2Complex/1
  HwModeRegister/1 -> MMul_dot_product/1
  HwModeRegister1/1 -> MMul_dot_product/2
  rd_7/1 -> MMul_dot_product_AC_minus_BD/1
  MMul_dot_product2/1 -> PipelineRegister2/1
  MMul_dot_product1/1 -> PipelineRegister1/1
  PipelineRegister2/1 -> MMul_dot_product_out_dtc2/1
  PipelineRegister3/1 -> MMul_dot_product_out_dtc3/1
  rd_15/1 -> MMul_dot_product_out_bypass/1(in0)
  PipelineRegister/1 -> MMul_dot_product_out_dtc/1
  MMul_dot_product_out_dtc1/1 -> rd_8/1
  rd_9/1 -> MMul_dot_product_AD_plus_BC/1
  MMul_dot_product_AD_plus_BC/1 -> MMul_dot_product_ReIm2Complex/2
  rd_13/1 -> tappedDelay/Enable
  tappedDelay/1(out0) -> rd_14/1
  rd_14/1 -> t/1
  MMul_dot_product_out_bypass/1(out0) -> t/2
  t/1 -> out0/1

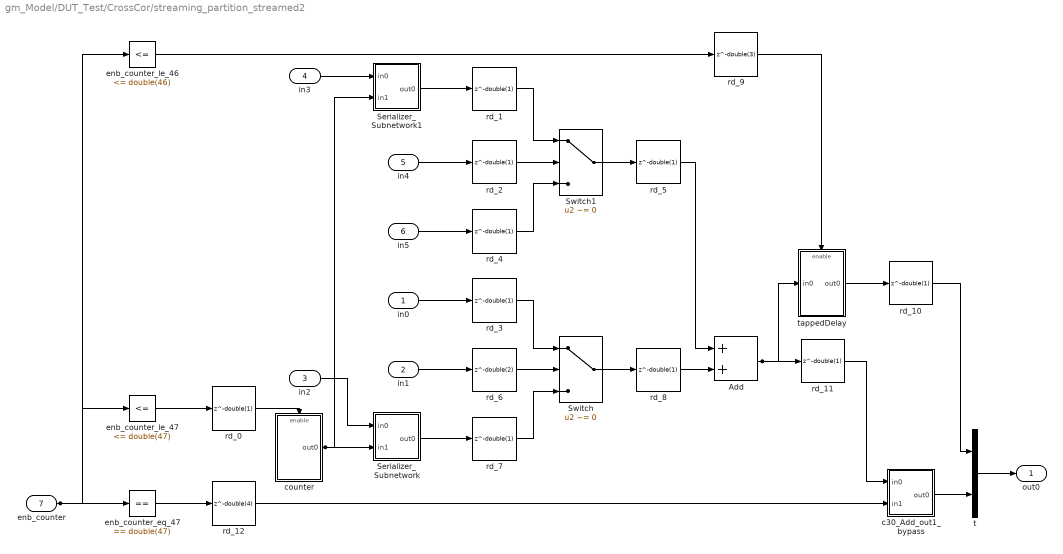
== system gm_Model/DUT_Test/CrossCor/streaming_partition_streamed2 ==
  in0 : Inport  OutDataTypeStr=fixdt(1, 18, 13)  SampleTime=3.125e-07
      settings: SignalType=complex
  in1 : Inport  Port=2  OutDataTypeStr=boolean  SampleTime=3.125e-07
  in2 : Inport  Port=3  OutDataTypeStr=fixdt(1, 18, 13)  PortDimensions=[2304 1]  SampleTime=3.125e-07
      settings: SignalType=complex
  in3 : Inport  Port=4  OutDataTypeStr=fixdt(1, 18, 13)  PortDimensions=[2304 1]  SampleTime=3.125e-07
      settings: SignalType=complex
  in4 : Inport  Port=5  OutDataTypeStr=boolean  SampleTime=3.125e-07
  in5 : Inport  Port=6  OutDataTypeStr=fixdt(1, 18, 13)  SampleTime=3.125e-07
      settings: SignalType=complex
  enb_counter : Inport  Port=7  OutDataTypeStr=uint16  SampleTime=3.125e-07
  Add : Sum  OutDataTypeStr=fixdt(1, 18, 13)  AccumDataTypeStr=fixdt(1, 18, 13)  SampleTime=3.125e-07
  Serializer_Subnetwork : Subsystem
  Serializer_Subnetwork1 : Subsystem
  Switch : Switch  Criteria=u2 ~= 0  Threshold="fi(0,0,1,0,\"hex\",\"0\")"  OutDataTypeStr=fixdt(1, 18, 13)  SampleTime=3.125e-07  SaturateOnIntegerOverflow=off  InputSameDT=off
  Switch1 : Switch  Criteria=u2 ~= 0  Threshold="fi(0,0,1,0,\"hex\",\"0\")"  OutDataTypeStr=fixdt(1, 18, 13)  SampleTime=3.125e-07  SaturateOnIntegerOverflow=off  InputSameDT=off
  c30_Add_out1_bypass : Subsystem
  counter : Subsystem
  enb_counter_eq_47 : simulink/Logic and Bit Operations/Compare To Constant  relop===  const=double(47)  OutDataTypeStr=boolean
  enb_counter_le_46 : simulink/Logic and Bit Operations/Compare To Constant  relop=<=  const=double(46)  OutDataTypeStr=boolean
  enb_counter_le_47 : simulink/Logic and Bit Operations/Compare To Constant  relop=<=  const=double(47)  OutDataTypeStr=boolean
  rd_{0..5,7..8,10..11} (10 alike) : Delay  DelayLength=double(1)  InitialCondition=0  SampleTime=3.125e-07
  rd_12 : Delay  DelayLength=double(4)  InitialCondition=0  SampleTime=3.125e-07
  rd_6 : Delay  DelayLength=double(2)  InitialCondition=0  SampleTime=3.125e-07
  rd_9 : Delay  DelayLength=double(3)  InitialCondition=0  SampleTime=3.125e-07
  t : Mux  Inputs=2
  tappedDelay : Subsystem
  out0 : Outport  OutDataTypeStr=fixdt(1, 18, 13)  PortDimensions=[2304 1]  SampleTime=3.125e-07
      settings: SignalType=complex
  wires:
  enb_counter_le_47/1 -> rd_0/1
  in5/1 -> rd_4/1
  enb_counter/1 -> enb_counter_eq_47/1, enb_counter_le_46/1, enb_counter_le_47/1
  rd_6/1 -> Switch/2
  enb_counter_le_46/1 -> rd_9/1
  enb_counter_eq_47/1 -> rd_12/1
  rd_9/1 -> tappedDelay/Enable
  rd_0/1 -> counter/Enable
  in3/1 -> Serializer_Subnetwork1/1(in0)
  rd_12/1 -> c30_Add_out1_bypass/2(in1)
  in1/1 -> rd_6/1
  in2/1 -> Serializer_Subnetwork/1(in0)
  counter/1(out0) -> Serializer_Subnetwork1/2(in1), Serializer_Subnetwork/2(in1)
  Serializer_Subnetwork1/1(out0) -> rd_1/1
  in4/1 -> rd_2/1
  in0/1 -> rd_3/1
  rd_3/1 -> Switch/1
  rd_4/1 -> Switch1/3
  Serializer_Subnetwork/1(out0) -> rd_7/1
  rd_1/1 -> Switch1/1
  t/1 -> out0/1
  rd_2/1 -> Switch1/2
  rd_5/1 -> Add/1
  rd_7/1 -> Switch/3
  Switch1/1 -> rd_5/1
  Switch/1 -> rd_8/1
  rd_8/1 -> Add/2
  Add/1 -> rd_11/1, tappedDelay/1(in0)
  tappedDelay/1(out0) -> rd_10/1
  rd_11/1 -> c30_Add_out1_bypass/1(in0)
  rd_10/1 -> t/1
  c30_Add_out1_bypass/1(out0) -> t/2

== system gm_Model/DUT_Test/CrossCor/streaming_partition_streamed3 ==
  in0 : Inport  OutDataTypeStr=fixdt(1, 18, 13)  PortDimensions=[2304 1]  SampleTime=3.125e-07
      settings: SignalType=complex
  in1 : Inport  Port=2  OutDataTypeStr=boolean  SampleTime=3.125e-07
  in2 : Inport  Port=3  OutDataTypeStr=fixdt(1, 18, 13)  PortDimensions=[2304 1]  SampleTime=3.125e-07
      settings: SignalType=complex
  enb_counter : Inport  Port=4  OutDataTypeStr=uint16  SampleTime=3.125e-07
  DataInSW : Switch  Criteria=u2 ~= 0  Threshold="fi(0,0,1,0,\"hex\",\"0\")"  OutDataTypeStr=fixdt(1, 18, 13)  SampleTime=3.125e-07  SaturateOnIntegerOverflow=off  InputSameDT=off
  Serializer_Subnetwork : Subsystem
  Serializer_Subnetwork1 : Subsystem
  c15_DataInSW_out1_bypass : Subsystem
  counter : Subsystem
  enb_counter_eq_47 : simulink/Logic and Bit Operations/Compare To Constant  relop===  const=double(47)  OutDataTypeStr=boolean
  enb_counter_le_46 : simulink/Logic and Bit Operations/Compare To Constant  relop=<=  const=double(46)  OutDataTypeStr=boolean
  enb_counter_le_47 : simulink/Logic and Bit Operations/Compare To Constant  relop=<=  const=double(47)  OutDataTypeStr=boolean
  rd_{0,2,5..6} (4 alike) : Delay  DelayLength=double(1)  InitialCondition=0  SampleTime=3.125e-07
  rd_1 : Delay  DelayLength=double(2)  InitialCondition=0  SampleTime=3.125e-07
  rd_3 : Delay  DelayLength=double(2)  InitialCondition=0  SampleTime=3.125e-07
  rd_4 : Delay  DelayLength=double(3)  InitialCondition=0  SampleTime=3.125e-07
  rd_7 : Delay  DelayLength=double(4)  InitialCondition=0  SampleTime=3.125e-07
  t : Mux  Inputs=2
  tappedDelay : Subsystem
  out0 : Outport  OutDataTypeStr=fixdt(1, 18, 13)  PortDimensions=[2304 1]  SampleTime=3.125e-07
      settings: SignalType=complex
  wires:
  enb_counter/1 -> enb_counter_eq_47/1, enb_counter_le_47/1, enb_counter_le_46/1
  in0/1 -> Serializer_Subnetwork/1(in0)
  enb_counter_le_46/1 -> rd_4/1
  rd_3/1 -> DataInSW/3
  rd_1/1 -> DataInSW/1
  counter/1(out0) -> Serializer_Subnetwork1/2(in1), Serializer_Subnetwork/2(in1)
  enb_counter_le_47/1 -> rd_0/1
  in2/1 -> Serializer_Subnetwork1/1(in0)
  enb_counter_eq_47/1 -> rd_7/1
  rd_0/1 -> counter/Enable
  rd_7/1 -> c15_DataInSW_out1_bypass/2(in1)
  Serializer_Subnetwork/1(out0) -> rd_1/1
  in1/1 -> rd_2/1
  Serializer_Subnetwork1/1(out0) -> rd_3/1
  rd_2/1 -> DataInSW/2
  rd_4/1 -> tappedDelay/Enable
  DataInSW/1 -> rd_6/1, tappedDelay/1(in0)
  tappedDelay/1(out0) -> rd_5/1
  rd_6/1 -> c15_DataInSW_out1_bypass/1(in0)
  rd_5/1 -> t/1
  c15_DataInSW_out1_bypass/1(out0) -> t/2
  t/1 -> out0/1
